simulink model "SimulatorSpencer"  (R2024a)
settings: Solver=VariableStepAuto  StartTime=0.0  StopTime=inf  MaxStep=1  RelTol=1e-5
model workspace (MAT data in the model file):
  A = 10
values from neighbouring files (symbols this model uses):
  CheckBox = modes(i)    [ACSModeSequence.m]    (also in Constants_gui.m = LampModes(i))
  I = [3000 0 0 ... (first row only)    [Constants_gui.m]    (also in constants.m; mbi.m = [15, .25, .20; set_up_HW7.m = I-Id; setupConstantRateSDA.m)
  invI = inv(I)    [Constants_gui.m]    (also in constants.m; mbi.m; set_up_HW7.m; setupConstantRateSDA.m)
  q_init = q_init/norm(q_init)    [Constants_gui.m]    (also in constants.m = [-0.5 -0.5 -0.5 0.5]; mbi.m = [0 0 0 1]'; set_up_HW7.m = [0 0 0 1]'; setupConstantRateSDA.m)
  wbn_init = pi/30*[0 0 0]'    [Constants_gui.m]    (also in constants.m = pi/180 * [0.1; 0.2; 0.15]; mbi.m = [0 0 0]'; set_up_HW7.m = pi/30*[0 0 .01]'; setupConstantRateSDA.m)
  wn = 0.01    [Constants_gui.m]    (also in constants.m = 0.05; setupConstantRateSDA.m = 0.05)
  zet = .7071    (= 0.7071)    [Constants_gui.m]    (also in constants.m; setupConstantRateSDA.m)
libraries: aerolibutil x9, sharedutil x8, sharedtransform x2, sldrtlib x1, dspinverses x1, vrlib x1
(part 1 of 4)
settings Model: Creator=nidhisonwalkar  LastModifiedBy=Spencer
settings SolverCC: DecoupledContinuousIntegration=on
settings DebuggingCC: SignalInfNanChecking=error  CheckMatrixSingularityMsg=error

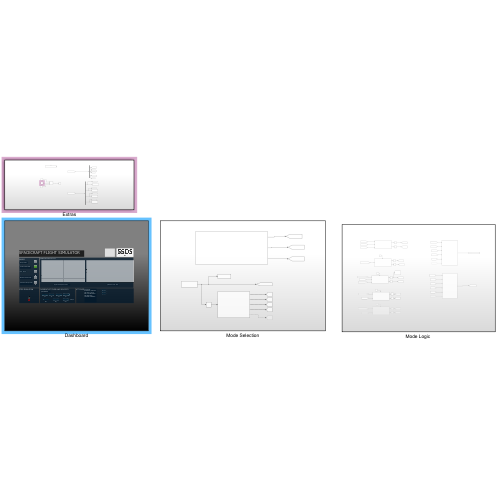
[thumbnail: Simulink's stored preview of the top-level diagram]
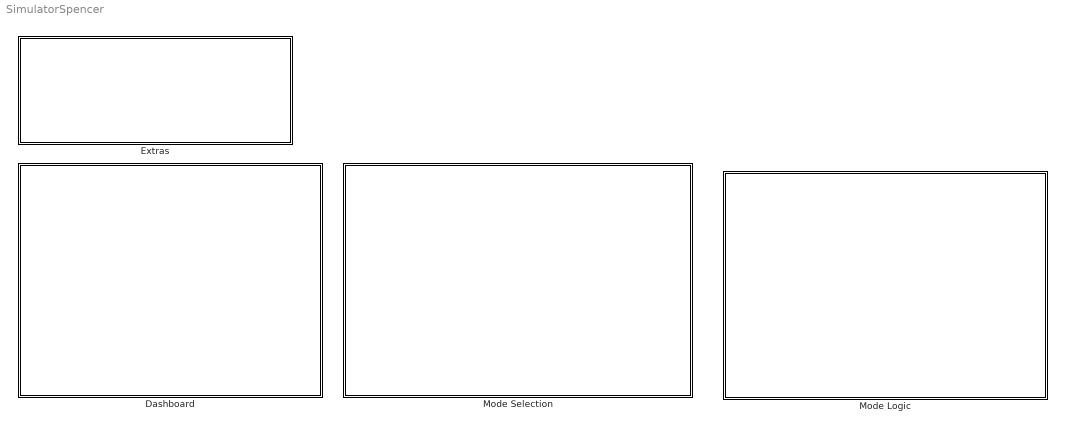
== system SimulatorSpencer ==
  Dashboard : Subsystem
  Extras : Subsystem
  "Mode Logic " : Subsystem
  Mode Selection : Subsystem

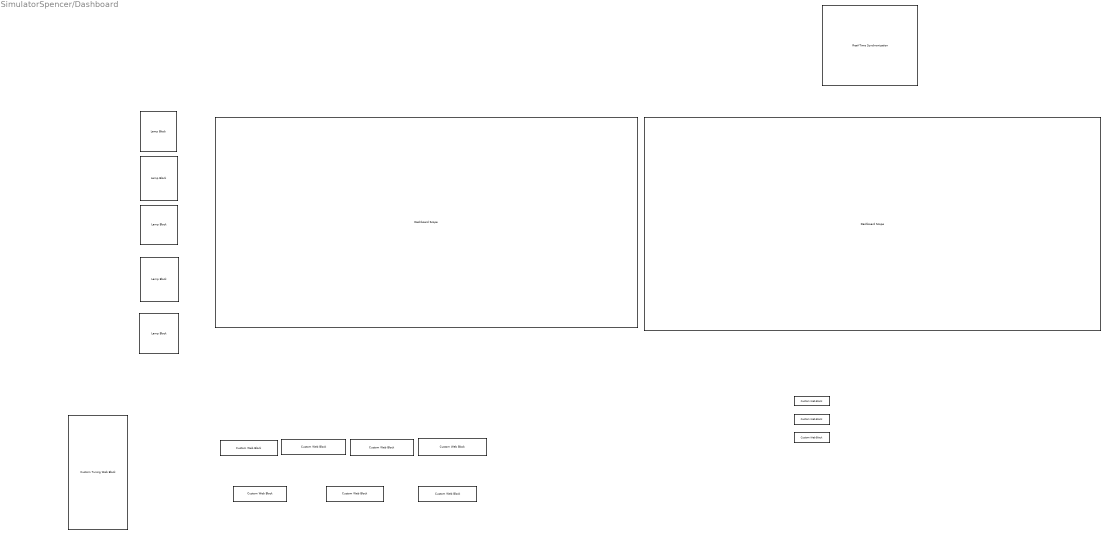
== system SimulatorSpencer/Dashboard ==
  note: SPACECRAFT FLIGHT SIMULATOR
  note: Constant Rate Mode
  note: Attitude Control Mode
  note: Startup Mode
  note: Momentum Dump Mode
  note: Slew Mode
  note: ATTITUDE
  note: ROLL
  note: PITCH
  note: YAW
  note: SIMULATION PLOTS
  note: MODES
  note: HRS
  note: MINS
  note: SECS
  note: QUATERNION
  note: CURRENT ATTITUDE AND VELOCITY
  note: VELOCITY
  note: RAD/S
  note: q1
  note: VELOCITY
  note: RAD/S
  note: q0
  note: q3
  note: q2
  note: QUATERNION
  note: Wx
  note: Wy
  note: Wz
  note: STOP SIMULATION
  note: Quaternion Over Time
  note: Angular Velocity Over Time
  note: ARTIFICIAL HORIZION, DISPLAYS FOR ROLL, PITCH, AND YAW REMOVED FOR NOW FOR TESTING PURPOSES
  Dashboard Scope1 : DashboardScope  LegendPosition=InsideTop  TicksPosition=Inside
  Dashboard Scope2 : DashboardScope  LegendPosition=InsideTop  TicksPosition=Inside
  Display{2,4..11} (9 alike) : CustomWebBlock  LabelPosition=Hide  ShowInitialText=on  Configuration="{\"components\":[{\"name\":\"DisplayComponent\",\"settings\":{\"bold\":false,\"font\":\"DSEG7 Classic\",\"fontColor\":[255,255,200],\"fontSize\":\"14\",\"format\":\"short\",\"formatString\":\"%d\",\"italic\":false,\"position\":[0,0,1,1],\"underline\":false}},{\"name\":\"BackgroundImageComponent\",\"settings\":{\"image\":{\"size\":[300,80],\"src\":\"data:image\\/svg+xml;base64,PHN2ZyBpZD0iZnJhbWUiIHhtbG5zPSJodHRwOi8vd3d3LnczLm9yZy8yMDAwL3N2ZyIgeG1sbnM6eGxpbms9Imh0dHA6Ly93d3cudzMub3JnLzE5OTkveGxpbmsiIHZpZXdCb3g9IjAgMCAzODAgMTAxIj48ZGVmcz48c3R5bGU+LmNscy0xe2ZpbGw6IzAwMmI0Mjt9LmNscy0ye2ZpbGw6IzQyNzA4Mjt9LmNscy0ze2ZpbGw6dXJsKCNyYWRpYWwtZ3JhZGllbnQpO308L3N0eWxlPjxyYWRpYWxHcmFkaWVudCBpZD0icmFkaWFsLWdyYWRpZW50IiBjeD0iMTkwIiBjeT0iNTAuNSIgcj0iMjY5LjIxIiBncmFkaWVudFVuaXRzPSJ1c2VyU3BhY2VPblVzZSI+PHN0b3Agb2Zmc2V0PSIwLjAxIiBzdG9wLWNvbG9yPSIjM2U0ZjU4Ii8+PHN0b3Agb2Zmc2V0PSIwLjA2IiBzdG9wLWNvbG9yPSIjNDQ1NzYxIi8+PHN0b3Agb2Zmc2V0PSIwLjE1IiBzdG9wLWNvbG9yPSIjNTU2YTc2Ii8+PHN0b3Agb2Zmc2V0PSIwLjI1IiBzdG9wLWNvbG9yPSIjNmQ4ODk1Ii8+PHN0b3Agb2Zmc2V0PSIwLjM4IiBzdG9wLWNvbG9yPSIjOGZiMmMzIi8+PHN0b3Agb2Zmc2V0PSIwLjUyIiBzdG9wLWNvbG9yPSIjYjZlNGZhIi8+PHN0b3Agb2Zmc2V0PSIxIiBzdG9wLWNvbG9yPSIjMTU0NjU3Ii8+PC9yYWRpYWxHcmFkaWVudD48L2RlZnM+PGcgaWQ9IkxheWVyXzIiIGRhdGEtbmFtZT0iTGF5ZXIgMiI+PGcgaWQ9IkxheWVyXzEtMiIgZGF0YS1uYW1lPSJMYXllciAxLTIiPjxyZWN0IGlkPSJyZWN0MTAzNiIgY2xhc3M9ImNscy0xIiB4PSIxMSIgeT0iMTEiIHdpZHRoPSIzNTgiIGhlaWdodD0iNzkiLz48cGF0aCBpZD0icGF0aDEwMzgiIGNsYXNzPSJjbHMtMiIgZD0iTTgsOFY5M0gzNzJWOFpNMzY5LDkwSDExVjExSDM2OVoiLz48cGF0aCBpZD0icGF0aDEwNDAiIGNsYXNzPSJjbHMtMyIgZD0iTTAsMFYxMDFIMzgwVjBaTTM3Miw5M0g4VjhIMzcyWiIvPjwvZz48L2c+PC9zdmc+\",\"srcOrientation\":\"Right\"},\"position\":[0,0,1,1],\"scaleMode\":\"0\"}},{\"name\":\"ForegroundImageComponent\",\"settings\":{\"angle\":0,\"image\":{\"size\":[0,0],\"src\":\"default\"},\"isForeground\":1,\"position\":[0,0,1,1],\"scaleMode\":\"0\"}}],\"settings\":{\"BindingType\":\"signal\",\"aspectRatio\":1.032258064516129,\"backgroundColor\":[0,0,0,\"1\"],\"backgroundOffset\":0.14,\"backgroundOpacity\":1,\"fixedAspectRatio\":\"on\",\"showBackgroundColor\":false,\"value\":0,\"version\":\"R2023b\"},\"type\":\"Display\"}"
  Lamp{,1..4} (5 alike) : LampBlock  LabelPosition=Hide
  Real-Time Synchronization : sldrtlib/Real-Time Synchronization  SampleTime=0.1  MaxMissedTicks=10  ShowMissedTicks=off  YieldWhenWaiting=off
  Toggle Switch : CustomTuningWebBlock  LabelPosition=Hide  ShowInitialText=on  Configuration="{\"components\":[{\"name\":\"CustomSwitchStateComponent\",\"settings\":{\"position\":[0,0,1,1],\"showAllLabels\":1,\"states\":[{\"HitRegion\":{\"position\":[0.5,0,1,0.5]},\"Image\":{\"position\":[0,0.24928571428571428,0.5014285714285714,1],\"size\":[0.5014285714285714,1],\"src\":\"data:image\\/svg+xml;base64,PHN2ZyB4bWxucz0iaHR0cDovL3d3dy53My5vcmcvMjAwMC9zdmciIHhtbG5zOnhsaW5rPSJodHRwOi8vd3d3LnczLm9yZy8xOTk5L3hsaW5rIiB2aWV3Qm94PSIwIDAgMzguMDQgMTUwIj48ZGVmcz48c3R5bGU+LmNscy0xe2ZpbGw6dXJsKCNyYWRpYWwtZ3JhZGllbnQpO30uY2xzLTJ7ZmlsbDp1cmwoI3JhZGlhbC1ncmFkaWVudC0yKTt9LmNscy0ze2ZpbGw6dXJsKCNXaGl0ZV9CbGFjayk7fS5jbHMtNHtmaWxsOnVybCgjcmFkaWFsLWdyYWRpZW50LTMpO30uY2xzLTV7ZmlsbDojNWI1YjViO30uY2xzLTZ7ZmlsbDp1cmwoI3Jh ...(+3556 chars)\",\"srcOrientation\":\"Right\"},\"Label\":{\"color\":[0.5019607843137255,0.5019607843137255,0.5019607843137255],\"icon\":{\"size\":[0,0],\"src\":[],\"srcOrientation\":\"Right\"},\"iconPlacement\":\"left\",\"opacity\":1,\"position\":[0.92,0.5],\"show\":true,\"text\":{\"content\":\"Off\",\"font\":\"Helvetica\",\"fontSize\":14}},\"Value\":0},{\"HitRegion\":{\"position\":[0,0,1,0.5]},\"Image\":{\"position\":[0,0.24928571428571428,0.5014285714285714,1],\"size\":[0.5014285714285714,1],\"src\":\"data:image\\/svg+xml;base64,PHN2ZyB4bWxucz0iaHR0cDovL3d3dy53My5vcmcvMjAwMC9zdmciIHhtbG5zOnhsaW5rPSJodHRwOi8vd3d3LnczLm9yZy8xOTk5L3hsaW5rIiB2aWV3Qm94PSIwIDAgMzguMDQgMTUwIj48ZGVmcz48c3R5bGU+LmNscy0xe2ZpbGw6dXJsKCNyYWRpYWwtZ3JhZGllbnQpO30uY2xzLTJ7ZmlsbDp1cmwoI3JhZGlhbC1ncmFkaWVudC0yKTt9LmNscy0ze2ZpbGw6dXJsKCNXaGl0ZV9CbGFjayk7fS5jbHMtNHtmaWxsOnVybCgjcmFkaWFsLWdyYWRpZW50LTMpO30uY2xzLTV7ZmlsbDojNWI1YjViO30uY2xzLTZ7ZmlsbDp1cmwoI3Jh ...(+3628 chars)\",\"srcOrientation\":\"Right\"},\"Label\":{\"color\":[0.5019607843137255,0.5019607843137255,0.5019607843137255],\"icon\":{\"size\":[0,0],\"src\":[],\"srcOrientation\":\"Right\"},\"iconPlacement\":\"left\",\"opacity\":1,\"position\":[0.08,0.5],\"show\":true,\"text\":{\"content\":\"On\",\"font\":\"Helvetica\",\"fontSize\":14}},\"Value\":1}]}},{\"name\":\"BackgroundImageComponent\",\"settings\":{\"image\":{\"size\":[70,135],\"src\":\"default\",\"srcOrientation\":\"Right\"},\"position\":[0,0,1,1],\"scaleMode\":\"0\"}},{\"name\":\"ForegroundImageComponent\",\"settings\":{\"image\":{\"size\":[0,0],\"src\":\"default\",\"srcOrientation\":[]},\"isForeground\":1,\"position\":[0,0,1,1],\"scaleMode\":\"0\"}}],\"settings\":{\"BindingType\":\"param\",\"backgroundColor\":[0,0,0],\"backgroundOffset\":0.14,\"fixedAspectRatio\":\"on\",\"foregroundColor\":[0,0,0],\"showBackgroundColor\":false,\"variant\":\"toggle\",\"version\":\"R2023a\"},\"type\":\"Switch\"}"
  YAW1 : CustomWebBlock  LabelPosition=Hide  ShowInitialText=on  Configuration="{\"components\":[{\"name\":\"DisplayComponent\",\"settings\":{\"bold\":false,\"font\":\"DSEG7 Classic\",\"fontColor\":[255,255,200],\"fontSize\":\"14\",\"format\":\"short\",\"formatString\":\"%d\",\"italic\":false,\"position\":[0,0,1,1],\"underline\":false}},{\"name\":\"BackgroundImageComponent\",\"settings\":{\"image\":{\"size\":[300,80],\"src\":\"data:image\\/svg+xml;base64,PHN2ZyBpZD0iZnJhbWUiIHhtbG5zPSJodHRwOi8vd3d3LnczLm9yZy8yMDAwL3N2ZyIgeG1sbnM6eGxpbms9Imh0dHA6Ly93d3cudzMub3JnLzE5OTkveGxpbmsiIHZpZXdCb3g9IjAgMCAzODAgMTAxIj48ZGVmcz48c3R5bGU+LmNscy0xe2ZpbGw6IzAwMmI0Mjt9LmNscy0ye2ZpbGw6IzQyNzA4Mjt9LmNscy0ze2ZpbGw6dXJsKCNyYWRpYWwtZ3JhZGllbnQpO308L3N0eWxlPjxyYWRpYWxHcmFkaWVudCBpZD0icmFkaWFsLWdyYWRpZW50IiBjeD0iMTkwIiBjeT0iNTAuNSIgcj0iMjY5LjIxIiBncmFkaWVudFVuaXRzPSJ1c2VyU3BhY2VPblVzZSI+PHN0b3Agb2Zmc2V0PSIwLjAxIiBzdG9wLWNvbG9yPSIjM2U0ZjU4Ii8+PHN0b3Agb2Zmc2V0PSIwLjA2IiBzdG9wLWNvbG9yPSIjNDQ1NzYxIi8+PHN0b3Agb2Zmc2V0PSIwLjE1IiBzdG9wLWNvbG9yPSIjNTU2YTc2Ii8+PHN0b3Agb2Zmc2V0PSIwLjI1IiBzdG9wLWNvbG9yPSIjNmQ4ODk1Ii8+PHN0b3Agb2Zmc2V0PSIwLjM4IiBzdG9wLWNvbG9yPSIjOGZiMmMzIi8+PHN0b3Agb2Zmc2V0PSIwLjUyIiBzdG9wLWNvbG9yPSIjYjZlNGZhIi8+PHN0b3Agb2Zmc2V0PSIxIiBzdG9wLWNvbG9yPSIjMTU0NjU3Ii8+PC9yYWRpYWxHcmFkaWVudD48L2RlZnM+PGcgaWQ9IkxheWVyXzIiIGRhdGEtbmFtZT0iTGF5ZXIgMiI+PGcgaWQ9IkxheWVyXzEtMiIgZGF0YS1uYW1lPSJMYXllciAxLTIiPjxyZWN0IGlkPSJyZWN0MTAzNiIgY2xhc3M9ImNscy0xIiB4PSIxMSIgeT0iMTEiIHdpZHRoPSIzNTgiIGhlaWdodD0iNzkiLz48cGF0aCBpZD0icGF0aDEwMzgiIGNsYXNzPSJjbHMtMiIgZD0iTTgsOFY5M0gzNzJWOFpNMzY5LDkwSDExVjExSDM2OVoiLz48cGF0aCBpZD0icGF0aDEwNDAiIGNsYXNzPSJjbHMtMyIgZD0iTTAsMFYxMDFIMzgwVjBaTTM3Miw5M0g4VjhIMzcyWiIvPjwvZz48L2c+PC9zdmc+\",\"srcOrientation\":\"Right\"},\"position\":[0,0,1,1],\"scaleMode\":\"0\"}},{\"name\":\"ForegroundImageComponent\",\"settings\":{\"angle\":0,\"image\":{\"size\":[0,0],\"src\":\"default\"},\"isForeground\":1,\"position\":[0,0,1,1],\"scaleMode\":\"0\"}}],\"settings\":{\"BindingType\":\"signal\",\"aspectRatio\":1.032258064516129,\"backgroundColor\":[0,0,0,\"1\"],\"backgroundOffset\":0.14,\"backgroundOpacity\":1,\"fixedAspectRatio\":\"on\",\"showBackgroundColor\":false,\"value\":0,\"version\":\"R2023b\"},\"type\":\"Display\"}"

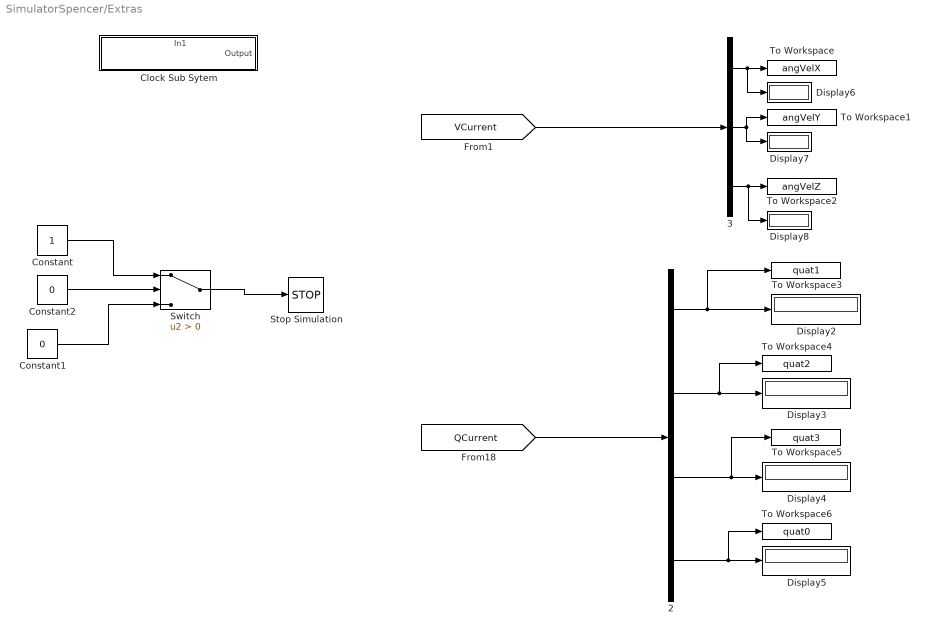
== system SimulatorSpencer/Extras ==
  " 2" : Demux
      settings: DisplayOption=none
  " 3" : Demux  Outputs=3
      settings: DisplayOption=none
  "Clock Sub Sytem " : Subsystem
      settings: PortSchema="{\"entries\":[{\"content\":{\"sides\":[{\"content\":{},\"type\":\"ConnectorPlacement.EquallySpacedRectSide\",\"uuid\":\"f28f70a2-a823-40ab-89bd-e0d8a2051dde\"},{\"content\":{\"connectorIds\":[\"Out1\"],\"side\":\"RIGHT\"},\"type\":\"ConnectorPlacement.EquallySpacedRectSide\",\"uuid\":\"5b03e72b-04aa-4879-9615-45db045b2acc\"},{\"content\":{\"connectorIds\":[\"In1\"],\"side\":\"TOP\"},\"type\":\"ConnectorPlacement.EquallySpacedRectSide\",\"uuid\":\"c7250e41-9a42-453a-a290-f4dbce75440c\"}]},\"type\":\"ConnectorPlacement.EquallySpacedConnector\",\"uuid\":\"7e9bb983-8bbf-43fa-9463-f14c417cdfdc\"}],\"packageUris\":[\"http://schema.mathworks.com/mf0/Connector/R2020b\"],\"version\":\"1.0\"}"
  Constant : Constant
  Constant1 : Constant  Value=0
  Constant2 : Constant  Value=0
  Display{2..8} (7 alike) : Display
  Stop Simulation : Stop
  Switch : Switch  Criteria=u2 > Threshold  SaturateOnIntegerOverflow=off  InputSameDT=off
  To Workspace : ToWorkspace  VariableName=angVelX  SaveFormat=Timeseries  SampleTime=-1
  To Workspace1 : ToWorkspace  VariableName=angVelY  SaveFormat=Timeseries  SampleTime=-1
  To Workspace2 : ToWorkspace  VariableName=angVelZ  SaveFormat=Timeseries  SampleTime=-1
  To Workspace3 : ToWorkspace  VariableName=quat1  SaveFormat=Timeseries  SampleTime=-1
  To Workspace4 : ToWorkspace  VariableName=quat2  SaveFormat=Timeseries  SampleTime=-1
  To Workspace5 : ToWorkspace  VariableName=quat3  SaveFormat=Timeseries  SampleTime=-1
  To Workspace6 : ToWorkspace  VariableName=quat0  SaveFormat=Timeseries  SampleTime=-1
  wires:
  " 2"/4 -> To Workspace6/1, Display5/1
  Switch/1 -> Stop Simulation/1
  [QCurrent] -> " 2"/1
  Constant1/1 -> Switch/3
  " 2"/1 -> To Workspace3/1, Display2/1
  " 3"/3 -> To Workspace2/1, Display8/1
  " 2"/3 -> To Workspace5/1, Display4/1
  " 3"/2 -> Display7/1, To Workspace1/1
  " 3"/1 -> Display6/1, To Workspace/1
  " 2"/2 -> To Workspace4/1, Display3/1
  Constant2/1 -> Switch/2
  [VCurrent] -> " 3"/1
  Constant/1 -> Switch/1

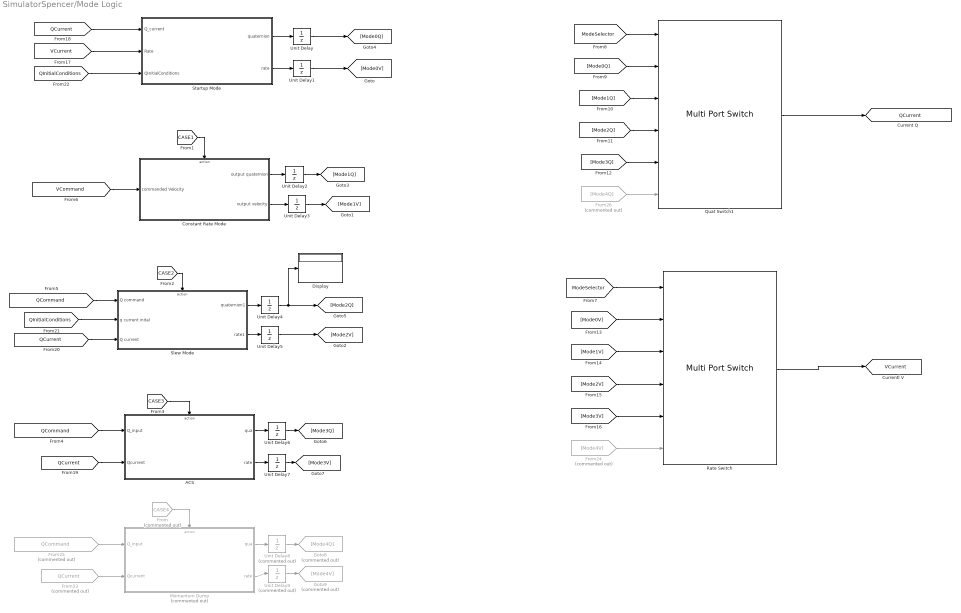
== system SimulatorSpencer/Mode Logic  ==
  ACS : Subsystem  TreatAsAtomicUnit=on
  Constant Rate Mode : Subsystem  TreatAsAtomicUnit=on
  Display : Display
  From : From  Commented=on  GotoTag=CASE4
  From23 : From  Commented=on  GotoTag=QCurrent  TagVisibility=global
  From24 : From  Commented=on  GotoTag=Mode4V
  From25 : From  Commented=on  GotoTag=QCommand  TagVisibility=global
  From26 : From  Commented=on  GotoTag=Mode4Q
  Goto8 : Goto  Commented=on  GotoTag=Mode4Q
  Goto9 : Goto  Commented=on  GotoTag=Mode4V
  Momentum Dump : Subsystem  Commented=on  TreatAsAtomicUnit=on
  Quat Switch1 : MultiPortSwitch  DataPortOrder=Specify indices  Inputs=6  DataPortIndices={0,1,2,3,4}  SaturateOnIntegerOverflow=off  InputSameDT=off
  Rate Switch : MultiPortSwitch  DataPortOrder=Specify indices  Inputs=6  DataPortIndices={0,1,2,3,4}  SaturateOnIntegerOverflow=off  InputSameDT=off
  Slew Mode : Subsystem  TreatAsAtomicUnit=on
  Startup Mode : Subsystem  TreatAsAtomicUnit=on
  Unit Delay{,1..7} (8 alike) : UnitDelay  SampleTime=-1  HasFrameUpgradeWarning=on
  Unit Delay8 : UnitDelay  Commented=on  SampleTime=-1  HasFrameUpgradeWarning=on
  Unit Delay9 : UnitDelay  Commented=on  SampleTime=-1  HasFrameUpgradeWarning=on
  tag scope: QCurrent=global, VCurrent=global
  wires:
  Startup Mode/2(rate) -> Unit Delay1/1
  Slew Mode/1(quaternion1) -> Unit Delay4/1
  [QCommand] -> ACS/1(Q_input)
  [QCommand] -> Slew Mode/1(Q command)
  [VCommand] -> Constant Rate Mode/1(commanded Velocity)
  Slew Mode/2(rate1) -> Unit Delay5/1
  Constant Rate Mode/2("output velocity ") -> Unit Delay3/1
  Constant Rate Mode/1(output quaternion) -> Unit Delay2/1
  Startup Mode/1(quaternion) -> Unit Delay/1
  ACS/1(qua) -> Unit Delay6/1
  ACS/2(rate) -> Unit Delay7/1
  [ModeSelector] -> Quat Switch1/1
  [ModeSelector] -> Rate Switch/1
  [Mode0Q] -> Quat Switch1/2
  [Mode1Q] -> Quat Switch1/3
  [Mode2Q] -> Quat Switch1/4
  [Mode3Q] -> Quat Switch1/5
  [Mode0V] -> Rate Switch/2
  [Mode1V] -> Rate Switch/3
  [Mode2V] -> Rate Switch/4
  [Mode3V] -> Rate Switch/5
  Quat Switch1/1 -> [QCurrent]
  Rate Switch/1 -> [VCurrent]
  [QCurrent] -> Startup Mode/1(Q_current)
  [VCurrent] -> Startup Mode/2(Rate)
  [QCurrent] -> ACS/2(Qcurrent)
  [QCurrent] -> Slew Mode/3(Q current)
  [QInitialConditions] -> Slew Mode/2("q current inital ")
  Unit Delay/1 -> [Mode0Q]
  Unit Delay1/1 -> [Mode0V]
  Unit Delay2/1 -> [Mode1Q]
  Unit Delay3/1 -> [Mode1V]
  Unit Delay4/1 -> [Mode2Q], Display/1
  Unit Delay5/1 -> [Mode2V]
  Unit Delay6/1 -> [Mode3Q]
  Unit Delay7/1 -> [Mode3V]
  [QInitialConditions] -> Startup Mode/3(QInitialConditions)
  From23/1 -> Momentum Dump/2(Qcurrent)
  Unit Delay8/1 -> Goto8/1
  From25/1 -> Momentum Dump/1(Q_input)
  Unit Delay9/1 -> Goto9/1
  Momentum Dump/2(rate) -> Unit Delay9/1
  Momentum Dump/1(qua) -> Unit Delay8/1
  From24/1 -> Rate Switch/6
  From26/1 -> Quat Switch1/6
  [CASE1] -> Constant Rate Mode/Action
  [CASE2] -> Slew Mode/Action
  [CASE3] -> ACS/Action
  From/1 -> Momentum Dump/Action

== system SimulatorSpencer/Mode Selection ==
  Commanded values : Subsystem
  Display : Display
  Goto8 : Goto  Commented=on  GotoTag=CASE4  TagVisibility=global
  Mode : Subsystem
  Switch Case : SwitchCase  CaseConditions={0,1, 2, 3, 4}  ShowDefaultCase=off
  Unit Delay : UnitDelay  SampleTime=-1  HasFrameUpgradeWarning=on
  tag scope: CASE0=global, CASE1=global, CASE2=global, CASE3=global, ModeSelector=global, QCommand=global, QInitialConditions=global, VCommand=global
  wires:
  Switch Case/4 -> [CASE3]
  Mode/1(Out1) -> Display/1, [ModeSelector], Unit Delay/1
  Switch Case/1 -> [CASE0]
  Switch Case/2 -> [CASE1]
  Switch Case/3 -> [CASE2]
  Commanded values/1(commanded quaternion) -> [QCommand]
  Commanded values/3(commanded Velocity) -> [VCommand]
  Unit Delay/1 -> Switch Case/1
  Commanded values/2(QInitialConditions) -> [QInitialConditions]
  Switch Case/5 -> Goto8/1

== system SimulatorSpencer/Extras/Clock Sub Sytem  ==
  In1 : Inport
  Clock : Clock
  Clock1 : Clock
  Clock2 : Clock
  Display : Display
  Display1 : Display
  Display2 : Display
  Gain : Gain
  Gain1 : Gain  Gain=3600
  Output : Outport
  wires:
  Gain1/1 -> Display2/1
  Clock/1 -> Output/1, Display/1
  Clock2/1 -> Gain/1
  Clock1/1 -> Gain1/1
  Gain/1 -> Display1/1

== system SimulatorSpencer/Mode Logic /ACS ==
  Q_input : Inport
  Qcurrent : Inport  Port=2
  Action Port : ActionPort  ActionPortLabel=case [ 3 ]:
  (q0,q1,q2,q3) to (q1,q2,q3,q0), : Subsystem
  "(q1,q2,q3,q0) to (q0,q1,q2,q3) " : Subsystem
  Add1 : Sum  Inputs=--
  Free Rigid Body 1 : Subsystem
  Kd1 : Gain  Gain=2 * zet * wn * I  Multiplication=Matrix(K*u)  SaturateOnIntegerOverflow=on  OutDataTypeStr=Inherit: Same as input  ParamDataTypeStr=Inherit: Same as input
  Kp1 : Gain  Gain=2 * wn^2 * I  Multiplication=Matrix(K*u)  SaturateOnIntegerOverflow=on  OutDataTypeStr=Inherit: Same as input  ParamDataTypeStr=Inherit: Same as input
  Quaternion Inverse1 : aerolibutil/Quaternion Inverse
  Quaternion Multiplication : aerolibutil/Quaternion Multiplication
  e_q_vect1 : Selector  InputPortWidth=4  IndexOptions=Index vector (dialog)  Indices=[1 2 3]  OutputSizes=1
  "w (q1,q2,q3,q0) to (q0,q1,q2,q3) " : Subsystem
      settings: PortSchema="{\"entries\":[{\"content\":{\"sides\":[{\"content\":{\"connectorIds\":[\"Out1\"]},\"type\":\"ConnectorPlacement.EquallySpacedRectSide\",\"uuid\":\"97b477ad-5663-4010-b344-d27b8ec095be\"},{\"content\":{\"connectorIds\":[\"In1\"],\"side\":\"RIGHT\"},\"type\":\"ConnectorPlacement.EquallySpacedRectSide\",\"uuid\":\"41fe4029-0263-4427-bdfc-3c26258b8a65\"},{\"content\":{\"side\":\"TOP\"},\"type\":\"ConnectorPlacement.EquallySpacedRectSide\",\"uuid\":\"9fb3a03d-539a-4245-bd7d-8174d3d0797f\"}]},\"type\":\"ConnectorPlacement.EquallySpacedConnector\",\"uuid\":\"44222554-f3ae-4bc6-b92c-7571a5ce84f7\"}],\"packageUris\":[\"http://schema.mathworks.com/mf0/Connector/R2020b\"],\"version\":\"1.0\"}"
  qua : Outport
  rate : Outport  Port=2
  wires:
  e_q_vect1/1 -> Kp1/1
  Kp1/1 -> Add1/1
  "(q1,q2,q3,q0) to (q0,q1,q2,q3) "/1(Out1) -> Quaternion Inverse1/1
  "w (q1,q2,q3,q0) to (q0,q1,q2,q3) "/1(Out1) -> Quaternion Multiplication/2
  Q_input/1 -> "(q1,q2,q3,q0) to (q0,q1,q2,q3) "/1(Q_input)
  Add1/1 -> Free Rigid Body 1/1(torque command)
  Quaternion Multiplication/1 -> (q0,q1,q2,q3) to (q1,q2,q3,q0),/1(In1)
  Kd1/1 -> Add1/2
  Qcurrent/1 -> "w (q1,q2,q3,q0) to (q0,q1,q2,q3) "/1(y)
  (q0,q1,q2,q3) to (q1,q2,q3,q0),/1(Out1) -> e_q_vect1/1
  Quaternion Inverse1/1 -> Quaternion Multiplication/1
  Free Rigid Body 1/1(q) -> qua/1
  Free Rigid Body 1/2(w) -> Kd1/1, rate/1

== system SimulatorSpencer/Mode Logic /Constant Rate Mode ==
  commanded Velocity : Inport
  Action Port : ActionPort  ActionPortLabel=case [ 1 ]:
  "Free Rigid Body " : Subsystem
  Kd1 : Gain  Gain=2 * zet * wn * I  Multiplication=Matrix(K*u)  SaturateOnIntegerOverflow=on  OutDataTypeStr=Inherit: Same as input  ParamDataTypeStr=Inherit: Same as input
  Sum1 : Sum  Inputs=|+-
  output quaternion : Outport
  "output velocity " : Outport  Port=2
  wires:
  Kd1/1 -> "Free Rigid Body "/1(In2)
  Sum1/1 -> Kd1/1
  commanded Velocity/1 -> Sum1/1
  "Free Rigid Body "/1(q) -> output quaternion/1
  "Free Rigid Body "/2(w) -> "output velocity "/1, Sum1/2

== system SimulatorSpencer/Mode Logic /Momentum Dump ==
  Q_input : Inport
  Qcurrent : Inport  Port=2
  Action Port : ActionPort  ActionPortLabel=case [ 3 ]:
  (q0,q1,q2,q3) to (q1,q2,q3,q0), : Subsystem
  "(q1,q2,q3,q0) to (q0,q1,q2,q3) " : Subsystem
  Add1 : Sum  Inputs=--
  Free Rigid Body 1 : Subsystem
  Kd1 : Gain  Gain=2 * zet * wn * I  Multiplication=Matrix(K*u)  SaturateOnIntegerOverflow=on  OutDataTypeStr=Inherit: Same as input  ParamDataTypeStr=Inherit: Same as input
  Kp1 : Gain  Gain=2 * wn^2 * I  Multiplication=Matrix(K*u)  SaturateOnIntegerOverflow=on  OutDataTypeStr=Inherit: Same as input  ParamDataTypeStr=Inherit: Same as input
  Quaternion Inverse1 : aerolibutil/Quaternion Inverse
  Quaternion Multiplication : aerolibutil/Quaternion Multiplication
  e_q_vect1 : Selector  InputPortWidth=4  IndexOptions=Index vector (dialog)  Indices=[1 2 3]  OutputSizes=1
  "w (q1,q2,q3,q0) to (q0,q1,q2,q3) " : Subsystem
      settings: PortSchema="{\"entries\":[{\"content\":{\"sides\":[{\"content\":{\"connectorIds\":[\"Out1\"]},\"type\":\"ConnectorPlacement.EquallySpacedRectSide\",\"uuid\":\"97b477ad-5663-4010-b344-d27b8ec095be\"},{\"content\":{\"connectorIds\":[\"In1\"],\"side\":\"RIGHT\"},\"type\":\"ConnectorPlacement.EquallySpacedRectSide\",\"uuid\":\"41fe4029-0263-4427-bdfc-3c26258b8a65\"},{\"content\":{\"side\":\"TOP\"},\"type\":\"ConnectorPlacement.EquallySpacedRectSide\",\"uuid\":\"9fb3a03d-539a-4245-bd7d-8174d3d0797f\"}]},\"type\":\"ConnectorPlacement.EquallySpacedConnector\",\"uuid\":\"44222554-f3ae-4bc6-b92c-7571a5ce84f7\"}],\"packageUris\":[\"http://schema.mathworks.com/mf0/Connector/R2020b\"],\"version\":\"1.0\"}"
  qua : Outport
  rate : Outport  Port=2
  wires:
  e_q_vect1/1 -> Kp1/1
  Kp1/1 -> Add1/1
  "(q1,q2,q3,q0) to (q0,q1,q2,q3) "/1(Out1) -> Quaternion Inverse1/1
  "w (q1,q2,q3,q0) to (q0,q1,q2,q3) "/1(Out1) -> Quaternion Multiplication/2
  Q_input/1 -> "(q1,q2,q3,q0) to (q0,q1,q2,q3) "/1(Q_input)
  Add1/1 -> Free Rigid Body 1/1(torque command)
  Quaternion Multiplication/1 -> (q0,q1,q2,q3) to (q1,q2,q3,q0),/1(In1)
  Kd1/1 -> Add1/2
  Qcurrent/1 -> "w (q1,q2,q3,q0) to (q0,q1,q2,q3) "/1(y)
  (q0,q1,q2,q3) to (q1,q2,q3,q0),/1(Out1) -> e_q_vect1/1
  Quaternion Inverse1/1 -> Quaternion Multiplication/1
  Free Rigid Body 1/1(q) -> qua/1
  Free Rigid Body 1/2(w) -> rate/1, Kd1/1

== system SimulatorSpencer/Mode Logic /Slew Mode ==
  Q command : Inport
  "q current inital " : Inport  Port=2
  Q current : Inport  Port=3
  Action Port : ActionPort  InitializeStates=reset  ActionPortLabel=case [ 2 ]:
  ACS : Subsystem
      settings: PortSchema="{\"entries\":[{\"content\":{\"sides\":[{\"content\":{\"connectorIds\":[\"Out3\",\"In1\",\"In2\",\"In3\"]},\"type\":\"ConnectorPlacement.EquallySpacedRectSide\",\"uuid\":\"9f52ffb6-d3dd-46bc-9b08-6a9b1eb08f5a\"},{\"content\":{\"connectorIds\":[\"Out1\",\"In4\",\"Out2\"],\"side\":\"RIGHT\"},\"type\":\"ConnectorPlacement.EquallySpacedRectSide\",\"uuid\":\"c36a10f6-7735-4632-825f-f5f96e6ba4a0\"},{\"content\":{\"side\":\"TOP\"},\"type\":\"ConnectorPlacement.EquallySpacedRectSide\",\"uuid\":\"f1931606-386a-4cfb-8b48-7eae19815e2a\"}]},\"type\":\"ConnectorPlacement.EquallySpacedConnector\",\"uuid\":\"335ce445-c3a9-4120-9c9c-ae8066099b2a\"}],\"packageUris\":[\"http://schema.mathworks.com/mf0/Connector/R2020b\"],\"version\":\"1.0\"}"
  DCM to Axis-Angle : Subsystem
  DCM to Axis-Angle3 : Subsystem
  For Loop : Subsystem
      settings: PortSchema="{\"entries\":[{\"content\":{\"sides\":[{\"content\":{\"connectorIds\":[\"In1\",\"In2\"]},\"type\":\"ConnectorPlacement.EquallySpacedRectSide\",\"uuid\":\"d1e910e7-02fe-476a-80f5-06936a5c67bc\"},{\"content\":{\"connectorIds\":[\"In4\",\"Out1\"],\"side\":\"RIGHT\"},\"type\":\"ConnectorPlacement.EquallySpacedRectSide\",\"uuid\":\"f2ee99f2-c038-4b18-8075-388ccc728d71\"},{\"content\":{\"connectorIds\":[\"In3\"],\"side\":\"TOP\"},\"type\":\"ConnectorPlacement.EquallySpacedRectSide\",\"uuid\":\"7923cf94-d68b-4fff-9236-03f2ad3fb038\"}]},\"type\":\"ConnectorPlacement.EquallySpacedConnector\",\"uuid\":\"859f0eee-a4bc-4454-90a5-75b168cd4378\"}],\"packageUris\":[\"http://schema.mathworks.com/mf0/Connector/R2020b\"],\"version\":\"1.0\"}"
  Subsystem : Subsystem
  quaternion1 : Outport
  rate1 : Outport  Port=2
  wires:
  DCM to Axis-Angle/1(Angle (phi)) -> For Loop/1(phi commanded)
  Q command/1 -> DCM to Axis-Angle3/1(Q_input)
  Subsystem/1(S value) -> For Loop/2(S value)
  "q current inital "/1 -> ACS/2(Q_input), DCM to Axis-Angle3/2(q current)
  DCM to Axis-Angle3/1(quatDiff) -> DCM to Axis-Angle/1(quatDiff)
  ACS/3(Output) -> For Loop/4(In4)
  DCM to Axis-Angle/2(Axis) -> ACS/3(axis), Subsystem/1(Axis)
  For Loop/1(Output) -> ACS/1(phi)
  Q current/1 -> ACS/4(Input)
  ACS/1(q) -> For Loop/3(phi value), quaternion1/1
  ACS/2(w) -> rate1/1

== system SimulatorSpencer/Mode Logic /Startup Mode ==
  Q_current : Inport
  Rate : Inport  Port=2
  QInitialConditions : Inport  Port=3
  Constant : Constant
  IC : InitialCondition  Value=[0;0;0;1]
  Switch : Switch  Criteria=u2 > Threshold  SaturateOnIntegerOverflow=off  InputSameDT=off
  quaternion : Outport
  rate : Outport  Port=2
  wires:
  QInitialConditions/1 -> Switch/1
  Constant/1 -> Switch/2
  Q_current/1 -> Switch/3
  Switch/1 -> IC/1
  Rate/1 -> rate/1
  IC/1 -> quaternion/1

== system SimulatorSpencer/Mode Selection/Commanded values ==
  Commanded Quaternion : Subsystem
  Commanded Quaternion1 : Subsystem
  Commanded Velocity : Subsystem
  commanded quaternion : Outport
  QInitialConditions : Outport  Port=2
  commanded Velocity : Outport  Port=3
  wires:
  Commanded Velocity/1(Out1) -> commanded Velocity/1
  Commanded Quaternion/1(Out1) -> commanded quaternion/1
  Commanded Quaternion1/1(QUaternion) -> QInitialConditions/1
